simulink model "sldemo_doublebounce"  (R2019b)
settings: Solver=ode23  StartTime=0.0  StopTime=42  MaxStep=0.01
undefined symbols (not defined in the file): ballBeep, dblBallaniminit
settings Model: ExtModeTrigMode=oneshot  ExtModeArmWhenConnect=off  ExtModeAutoUpdateStatusClock=off  Creator=The MathWorks, Inc.  LastModifiedBy=bhisma
settings SolverCC: ConsecutiveZCsStepRelTol=1e-7  MaxConsecutiveZCs=10  ZeroCrossAlgorithm=Adaptive
settings DataIOCC: ExternalInput=[]  InitialState=[]  SaveFormat=StructureWithTime  SaveOutput=off  SignalLogging=off  SaveTime=off  OutputTimes="[3.81818      7.63636      11.4545      15.2727      19.0909      22.9091      26.7273      30.5455      34.3636      38.1818]"
settings OptimizationCC: DefaultParameterBehavior=Inlined  InlineInvariantSignals=on  ExpressionDepthLimit=2147483647  InitFltsAndDblsToZero=on  EfficientFloat2IntCast=on  LifeSpan=inf
settings DebuggingCC: SaveWithParameterizedLinksMsg=none  UnderspecifiedInitializationDetection=Classic  MergeDetectMultiDrivingBlocksExec=none  MultiTaskDSMMsg=warning  MultiTaskCondExecSysMsg=none  FcnCallInpInsideContextMsg=warning  StateNameClashWarn=warning  SFUnexpectedBacktrackingDiag=warning  SFNoUnconditionalDefaultTransitionDiag=warning  SFExecutionAtInitializationDiag=none  ArithmeticOperatorsInVariantConditions=warning
settings HardwareCC: ProdBitPerPointer=32  ProdBitPerSizeT=32  ProdBitPerPtrDiffT=32  ProdLargestAtomicFloat=None  ProdIntDivRoundTo=Undefined  ProdEndianess=Unspecified  ProdWordSize=32  ProdHWDeviceType=32-bit Generic  TargetBitPerLong=64  TargetBitPerPointer=64  TargetBitPerSizeT=64  TargetBitPerPtrDiffT=64  TargetLongLongMode=on  TargetIntDivRoundTo=Zero  TargetEndianess=LittleEndian  TargetWordSize=64  TargetHWDeviceType=MATLAB Host  ProdEqTarget=off
settings ModelReferenceCC: PropagateSignalLabelsOutOfModel=off
settings SFSimCC: SimUseLocalCustomCode=off  CustomCodeUndefinedFunction=UseInterfaceOnly
settings RTWCC: Description=Rapid Simulation Target  SystemTargetFile=rsim.tlc  TemplateMakefile=rsim_default_tmf  RetainRTWFile=on  TLCAssert=on  RTWUseLocalCustomCode=off
settings CodeAppCC: StateflowObjectComments=on
settings RSimTargetCC: TargetFcnLib=ansi_tfl_tmw.mat  PreserveStateflowLocalDataDimensions=off
settings ConfigComp: CovMetricSettings=d  CovHtmlReporting=on  CovSaveCumulativeToWorkspaceVar=on  CovSaveSingleToWorkspaceVar=on  CovExternalEMLEnable=off

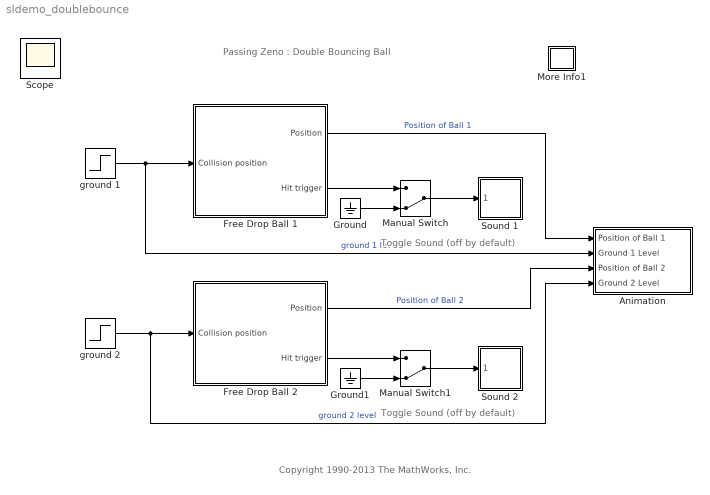
== system sldemo_doublebounce ==
  note: Passing Zeno : Double Bouncing Ball
  note: Copyright 1990-2013 The MathWorks, Inc.
  note: Toggle Sound
      | (off by default)
  note: Toggle Sound
      | (off by default)
  Animation : Subsystem  LoadFcn=dblBallaniminit;
      settings: ModelCloseFcn=|
      | dblbncfig = get_param(gcb,'UserData');
      | if (isfield(dblbncfig,'figure') && ishghandle(dblbncfig.figure,'figure'))
      |    close(dblbncfig.figure);
      | end
      | clear dblbncfig;
  Free Drop Ball 1 : Subsystem  mask{x0=30, v0=14}
      mask prompts: x0 "Initial position"; v0 "Initial speed"
      mask Display:
      | port_label('output', 1, 'Position')
      | port_label('output', 2, 'Hit trigger')
      | port_label('input', 1, 'Collision position')
  Free Drop Ball 2 : Subsystem  mask{x0=30, v0=25}
      mask prompts: x0 "Initial position"; v0 "Initial speed"
      mask Display:
      | port_label('output', 1, 'Position')
      | port_label('output', 2, 'Hit trigger')
      | port_label('input', 1, 'Collision position')
  Ground : Ground
  Ground1 : Ground
  Manual Switch : ManualSwitch  CurrentSetting=0
  Manual Switch1 : ManualSwitch  CurrentSetting=0
  More Info1 : Subsystem
      settings: OpenFcn=showExample('simulink_general/sldemo_doublebounceExample')
      mask Display: disp('?')
  Sound 1 : Subsystem  mask{delay=0.5}
      mask prompts: delay "Sound Delay(0-1. 0 Disable)"
      mask help: This block simulates the sound when the ball hit the ground. When the delay parameter is set to 0, it will disable the sound. Adjust this parameter if the sound is not clear.
      mask Display: disp('Sound')
  Sound 2 : Subsystem  mask{delay=0.5}
      mask prompts: delay "Sound Delay(0-1. 0 Disable)"
      mask help: This block simulates the sound when the ball hit the ground. When the delay parameter is set to 0, it will disable the sound. Adjust this parameter if the sound is not clear.
      mask Display: disp('Sound')
  ground 1 : Step  Time=20  Before=30  After=10  SampleTime=0
  ground 2 : Step  Time=25  Before=30  After=10  SampleTime=0
  Scope : Scope
  wires:
  ground 1/1 -> Free Drop Ball 1/1(Collision position), Animation/2(Ground 1 Level)  "ground 1 level"
  ground 2/1 -> Free Drop Ball 2/1(Collision position), Animation/4(Ground 2 Level)  "ground 2 level"
  Free Drop Ball 1/1(Position) -> Animation/1(Position of Ball 1)  "Position of Ball 1"
  Free Drop Ball 2/1(Position) -> Animation/3(Position of Ball 2)  "Position of Ball 2"
  Manual Switch/1 -> Sound 1/1(trigger)
  Free Drop Ball 1/2(Hit trigger) -> Manual Switch/1
  Ground/1 -> Manual Switch/2
  Manual Switch1/1 -> Sound 2/1(trigger)
  Free Drop Ball 2/2(Hit trigger) -> Manual Switch1/1
  Ground1/1 -> Manual Switch1/2

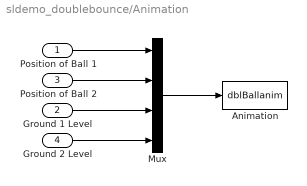
== system sldemo_doublebounce/Animation ==
  Position of Ball 1 : Inport
  Ground 1 Level : Inport  Port=2
  Position of Ball 2 : Inport  Port=3
  Ground 2 Level : Inport  Port=4
  "Animation " : S-Function  FunctionName=dblBallanim  Parameters=ts, y0  SFunctionDeploymentMode=off  EnableBusSupport=off  mask{ts=0.01, y0=[30 30 30 30]}
      mask prompts: ts "Sample Time (< 0)"; y0 "Initial position"
      mask help: This block animate the simulation results. Increase the sample time if the simulation is too slow.
  Mux : Mux
  wires:
  Mux/1 -> "Animation "/1
  Position of Ball 1/1 -> Mux/1
  Position of Ball 2/1 -> Mux/2
  Ground 1 Level/1 -> Mux/3
  Ground 2 Level/1 -> Mux/4

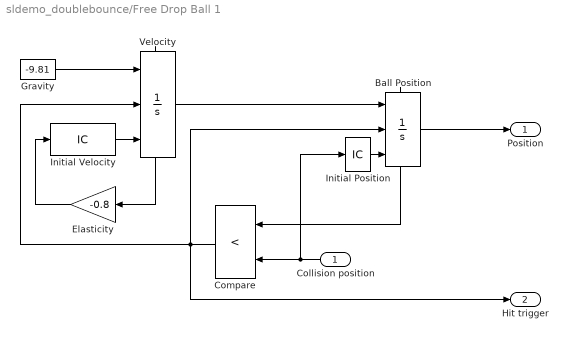
== system sldemo_doublebounce/Free Drop Ball 1 ==
  Collision position : Inport
  "Ball Position " : Integrator  ExternalReset=rising  InitialConditionSource=external  LowerSaturationLimit=-eps  ShowStatePort=on  ZeroCross=off
  Compare : RelationalOperator  Operator=<  OutDataTypeStr=boolean  RndMeth=Nearest  InputSameDT=on
  Elasticity : Gain  Gain=-0.8  SaturateOnIntegerOverflow=on  OutDataTypeStr=Inherit: Same as input  ParamDataTypeStr=Inherit: Same as input
  Gravity : Constant  Value=-9.81
  Initial Position : InitialCondition  Value=x0
  Initial Velocity : InitialCondition  Value=v0
  Velocity : Integrator  ExternalReset=rising  InitialConditionSource=external  ShowStatePort=on
  Position : Outport  VectorParamsAs1DForOutWhenUnconnected=off
  Hit trigger : Outport  Port=2  VectorParamsAs1DForOutWhenUnconnected=off
  wires:
  Velocity/State -> Elasticity/1
  Initial Velocity/1 -> Velocity/3
  Elasticity/1 -> Initial Velocity/1
  Velocity/1 -> "Ball Position "/1
  Gravity/1 -> Velocity/1
  Compare/1 -> Velocity/2, "Ball Position "/2, Hit trigger/1
  "Ball Position "/State -> Compare/1
  Collision position/1 -> Initial Position/1, Compare/2
  Initial Position/1 -> "Ball Position "/3
  "Ball Position "/1 -> Position/1

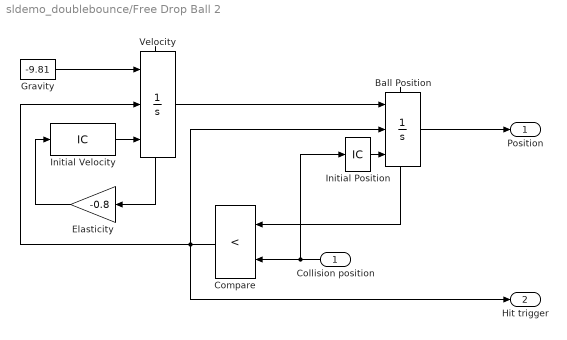
== system sldemo_doublebounce/Free Drop Ball 2 ==
  Collision position : Inport
  "Ball Position " : Integrator  ExternalReset=rising  InitialConditionSource=external  LowerSaturationLimit=-eps  ShowStatePort=on  ZeroCross=off
  Compare : RelationalOperator  Operator=<  OutDataTypeStr=boolean  RndMeth=Nearest  InputSameDT=on
  Elasticity : Gain  Gain=-0.8  SaturateOnIntegerOverflow=on  OutDataTypeStr=Inherit: Same as input  ParamDataTypeStr=Inherit: Same as input
  Gravity : Constant  Value=-9.81
  Initial Position : InitialCondition  Value=x0
  Initial Velocity : InitialCondition  Value=v0
  Velocity : Integrator  ExternalReset=rising  InitialConditionSource=external  ShowStatePort=on
  Position : Outport  VectorParamsAs1DForOutWhenUnconnected=off
  Hit trigger : Outport  Port=2  VectorParamsAs1DForOutWhenUnconnected=off
  wires:
  Velocity/State -> Elasticity/1
  Initial Velocity/1 -> Velocity/3
  Elasticity/1 -> Initial Velocity/1
  Velocity/1 -> "Ball Position "/1
  Gravity/1 -> Velocity/1
  Compare/1 -> Velocity/2, "Ball Position "/2, Hit trigger/1
  "Ball Position "/State -> Compare/1
  Collision position/1 -> Initial Position/1, Compare/2
  Initial Position/1 -> "Ball Position "/3
  "Ball Position "/1 -> Position/1

== system sldemo_doublebounce/More Info1 ==

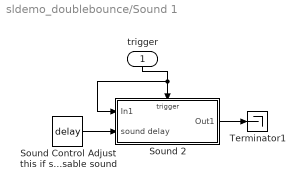
== system sldemo_doublebounce/Sound 1 ==
  trigger : Inport
  Sound 2 : Subsystem  TreatAsAtomicUnit=on
  Sound Control Adjust this if sound is not good. =0  Disable sound : Constant  Value=delay
  Terminator1 : Terminator
  wires:
  Sound Control Adjust this if sound is not good. =0  Disable sound/1 -> Sound 2/2(sound delay)
  Sound 2/1(Out1) -> Terminator1/1
  trigger/1 -> Sound 2/Trigger, Sound 2/1(In1)

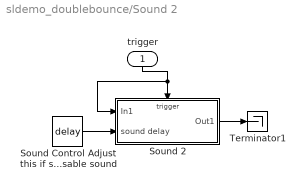
== system sldemo_doublebounce/Sound 2 ==
  trigger : Inport
  Sound 2 : Subsystem  TreatAsAtomicUnit=on
  Sound Control Adjust this if sound is not good. =0  Disable sound : Constant  Value=delay
  Terminator1 : Terminator
  wires:
  Sound Control Adjust this if sound is not good. =0  Disable sound/1 -> Sound 2/2(sound delay)
  Sound 2/1(Out1) -> Terminator1/1
  trigger/1 -> Sound 2/Trigger, Sound 2/1(In1)

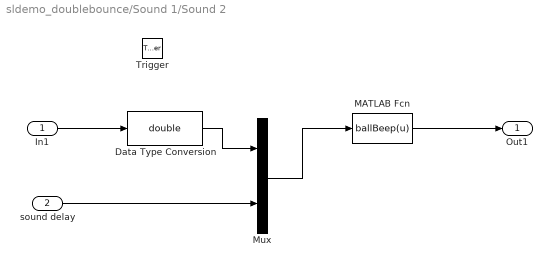
== system sldemo_doublebounce/Sound 1/Sound 2 ==
  In1 : Inport
  sound delay : Inport  Port=2
  Trigger : TriggerPort  VariantControl=Variant
  Data Type Conversion : DataTypeConversion  OutDataTypeStr=double
  MATLAB Fcn : MATLABFcn  MATLABFcn=ballBeep(u)
  Mux : Mux  Inputs=2
  Out1 : Outport  VectorParamsAs1DForOutWhenUnconnected=off
  wires:
  In1/1 -> Data Type Conversion/1
  MATLAB Fcn/1 -> Out1/1
  Data Type Conversion/1 -> Mux/1
  sound delay/1 -> Mux/2
  Mux/1 -> MATLAB Fcn/1

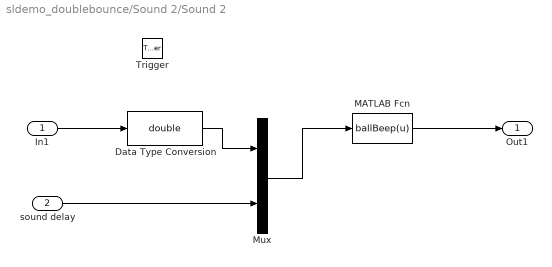
== system sldemo_doublebounce/Sound 2/Sound 2 ==
  In1 : Inport
  sound delay : Inport  Port=2
  Trigger : TriggerPort  VariantControl=Variant
  Data Type Conversion : DataTypeConversion  OutDataTypeStr=double
  MATLAB Fcn : MATLABFcn  MATLABFcn=ballBeep(u)
  Mux : Mux  Inputs=2
  Out1 : Outport  VectorParamsAs1DForOutWhenUnconnected=off
  wires:
  In1/1 -> Data Type Conversion/1
  MATLAB Fcn/1 -> Out1/1
  Data Type Conversion/1 -> Mux/1
  sound delay/1 -> Mux/2
  Mux/1 -> MATLAB Fcn/1
